simulink model "unicycle_polar_simulink"  (R2020b)
settings: Solver=VariableStepAuto  StartTime=0.0  StopTime=10.0  RelTol=1e-3
libraries: robotmobilelib x1, simulink x1
settings Model: Creator=nijil  LastModifiedBy=nijil

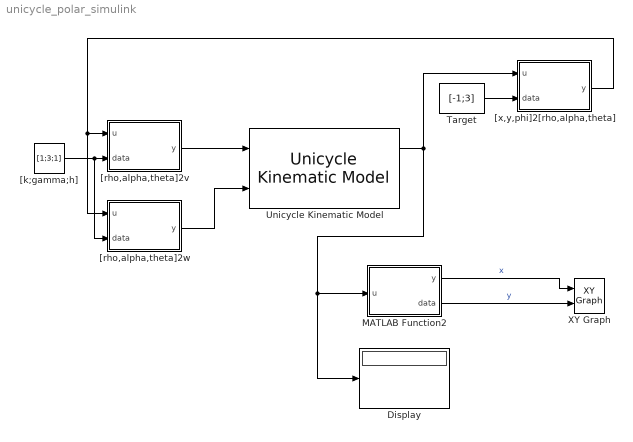
== system unicycle_polar_simulink ==
  Display : Display
  MATLAB Function2 : MATLAB Function  TreatAsAtomicUnit=on
  Target : Constant  Value=[-1;3]  VectorParams1D=off
  Unicycle Kinematic Model : robotmobilelib/Unicycle Kinematic Model  VehicleInputs=Vehicle Speed & Heading Angular Velocity  WheelRadius=0.1  WheelSpeedRange=[-Inf Inf]  InitialState=initial_state  SimulateUsing=Interpreted execution
      settings: SourceProductBaseCode=RO
  XY Graph : simulink/Sinks/XY Graph  xmin=-5  xmax=5  ymin=-5  ymax=5  st=-1
  "[k;gamma;h]" : Constant  Value=[1;3;1]  VectorParams1D=off
  "[rho,alpha,theta]2v" : MATLAB Function  TreatAsAtomicUnit=on
  "[rho,alpha,theta]2w" : MATLAB Function  TreatAsAtomicUnit=on
  "[x,y,phi]2[rho,alpha,theta]" : MATLAB Function  TreatAsAtomicUnit=on
  wires:
  "[rho,alpha,theta]2v"/1(y) -> Unicycle Kinematic Model/1
  Unicycle Kinematic Model/1 -> "[x,y,phi]2[rho,alpha,theta]"/1(u), Display/1, MATLAB Function2/1(u)
  "[k;gamma;h]"/1 -> "[rho,alpha,theta]2w"/2(data), "[rho,alpha,theta]2v"/2(data)
  "[rho,alpha,theta]2w"/1(y) -> Unicycle Kinematic Model/2
  MATLAB Function2/1(y) -> XY Graph/1  "x"
  MATLAB Function2/2(data) -> XY Graph/2  "y"
  Target/1 -> "[x,y,phi]2[rho,alpha,theta]"/2(data)
  "[x,y,phi]2[rho,alpha,theta]"/1(y) -> "[rho,alpha,theta]2w"/1(u), "[rho,alpha,theta]2v"/1(u)

== matlab function unicycle_polar_simulink/[rho,alpha,theta]2v ==
  data: u input; y output; data input
function y = fcn(u, data)
%data=[k;gamma;h], u=[rho,alpha,theta]

y = data(2)*cos(u(2))*u(1);

== matlab function unicycle_polar_simulink/MATLAB Function2 ==
  data: u input; y output; data output
function [y,data] = fcn(u)
y=u(1);
data = u(2);

== matlab function unicycle_polar_simulink/[x,y,phi]2[rho,alpha,theta] ==
  data: u input; y output; data input
function y = fcn(u, data)
%u=[x;y;phi], data=[x_c;y_c], y=[rho,alpha,theta]
rho=sqrt((u(1)-data(1))^2+(u(2)-data(2))^2);
alpha=-u(3)+atan2((data(2)-u(2)),(data(1)-u(1)));
theta=atan2((data(2)-u(2)),(data(1)-u(1)));
y =[rho;alpha;theta];

== matlab function unicycle_polar_simulink/[rho,alpha,theta]2w ==
  data: u input; y output; data input
function y = fcn(u, data)
%data=[k;gamma;h], u=[rho,alpha,theta]
y =data(1)*u(2)+data(2)*cos(u(2))*sin(u(2))*(u(2)+data(3)*u(3))/u(2);
